simulink model "Example_2_1ODE"  (Simulink 7.4)
settings: Solver=ode45  StartTime=0.0  StopTime=10.0  RelTol=1e-3
settings Model: Creator=David  LastModifiedBy=David
settings DebuggingCC: StrictBusMsg=ErrorLevel1

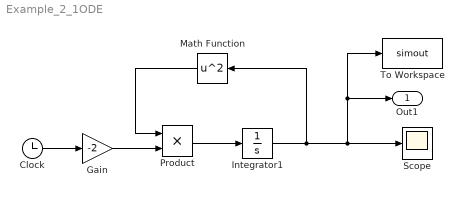
== system Example_2_1ODE ==
  Clock : Clock
      settings: Decimation=10
  Gain : Gain  Gain=-2
  Integrator1 : Integrator  InitialCondition=.5
  Math Function : Math  Operator=square  SaturateOnIntegerOverflow=on
  Product : Product  RndMeth=Zero
  Scope : Scope
  To Workspace : ToWorkspace  VariableName=simout  SampleTime=-1  SaveFormat=Structure
  Out1 : Outport
  wires:
  Integrator1/1 -> Scope/1, Out1/1, To Workspace/1, Math Function/1
  Clock/1 -> Gain/1
  Product/1 -> Integrator1/1
  Math Function/1 -> Product/1
  Gain/1 -> Product/2
